simulink model "spring_mass_model_01"  (R2014a)
settings: Solver=FixedStepDiscrete  StartTime=0.0  StopTime=inf  FixedStep=sample_time  RelTol=1e-3
values from neighbouring files (symbols this model uses):
  g = g_real    (= 9.803)    [max_motor_torques.m]
  l0_leg = 0.97    [max_motor_torques.m]
  l0_virtual = sqrt(d^2+l0_leg^2-2*d*l0_leg*cos(phi0))    [max_motor_torques.m]
undefined symbols (not defined in the file or in its folder): alpha_apex, alpha_max, alpha_min, boom_mount_angle, c_energy, contact_threshold, control_start_time, d_y_boom_com_offset, d_y_boom_hip_offset, d_y_com, d_y_mount_to_com, desired_torso_angle, DiscIntNeverNeededParam, dt_thrust, dx_avg_desired, extra_leg_damping, F_thrust, fcut_contact, ff_energy_l, ff_energy_r, g_reduced, h_boom, i_limit_lateral, i_robot, initial_com_height, initial_dt, initial_dx, j_leg, j_rotor, j_segments, k0_virtual, k_placement, k_sea, kd_flight, kd_lateral, kd_leg_angle, kd_motor, kd_raibert, kd_torso, ki_lateral, kp_flight_max, kp_flight_min, kp_lateral, kp_leg_angle, kp_motor, kp_raibert, kp_torso, l0_max_angle_error, l0_min_angle_error, l0_min_flight_time, l_boom, l_boom_projected, l_max, l_min, l_retract_escape, l_retract_swing, l_seg, lambda1, lambda2, lateral_offset ... (+33)
libraries: simulink x22, simulink_extras x2
(part 2 of 3)

== system spring_mass_model_01/Control/Behavior Control/Contact Estimation/Contact Time ==
  Enable : EnablePort  StatesWhenEnabling=reset  ShowOutputPort=on
  Constant : Constant
  Discrete-Time Integrator : DiscreteIntegrator  IntegratorMethod=Accumulation: Forward Euler  gainval=sample_time  ExternalReset=rising  SampleTime=sample_time  ICPrevOutput=DiscIntNeverNeededParam  ICPrevScaledInput=DiscIntNeverNeededParam
  ts [s] : Outport  InitialOutput=[0]
  wires:
  Constant/1 -> Discrete-Time Integrator/1
  Enable/1 -> Discrete-Time Integrator/2
  Discrete-Time Integrator/1 -> ts [s]/1

== system spring_mass_model_01/Control/Behavior Control/Contact Estimation/Last Contact Time ==
  ts [s] : Inport
  Trigger : TriggerPort  TriggerType=falling  PortDimensions=1
  Ts [s] : Outport  InitialOutput=[initial_dt]
  wires:
  ts [s]/1 -> Ts [s]/1

== system spring_mass_model_01/Control/Behavior Control/Contact Estimation/Leg Torque Measurements ==
  q : Inport
  Right/Left Stance [1/0] : Inport  Port=2
  Spring Stiffness3 : Gain  Gain=k_sea(1)
  Spring Stiffness4 : Gain  Gain=k_sea(3)
  Spring Stiffness5 : Gain  Gain=k_sea(2)
  Spring Stiffness6 : Gain  Gain=k_sea(4)
  Sum{1..3,6} (4 alike) : Sum  Inputs=-+|
  Switch : Switch  Criteria=u2 ~= 0
  Switch1 : Switch  Criteria=u2 ~= 0
  backGearL : Selector  InputPortWidth=13  Indices=[6]
  backGearR : Selector  InputPortWidth=13  Indices=[2]
  backJointL : Selector  InputPortWidth=13  Indices=[5]
  backJointR : Selector  InputPortWidth=13  Indices=[1]
  frontGearL : Selector  InputPortWidth=13  Indices=[8]
  frontGearR : Selector  InputPortWidth=13  Indices=[4]
  frontJointL : Selector  InputPortWidth=13  Indices=[7]
  frontJointR : Selector  InputPortWidth=13  Indices=[3]
  Back [Nm] : Outport
  Front [Nm] : Outport  Port=2
  wires:
  Spring Stiffness6/1 -> Switch/3
  Spring Stiffness5/1 -> Switch/1
  Spring Stiffness4/1 -> Switch1/3
  Spring Stiffness3/1 -> Switch1/1
  q/1 -> backJointR/1, frontGearL/1, frontJointL/1, frontGearR/1, frontJointR/1, backGearL/1, backJointL/1, backGearR/1
  backGearR/1 -> Sum6/2
  frontJointR/1 -> Sum1/1
  frontGearR/1 -> Sum1/2
  backJointR/1 -> Sum6/1
  Switch/1 -> Front [Nm]/1
  Sum1/1 -> Spring Stiffness5/1
  Sum6/1 -> Spring Stiffness3/1
  backGearL/1 -> Sum2/2
  frontJointL/1 -> Sum3/1
  frontGearL/1 -> Sum3/2
  backJointL/1 -> Sum2/1
  Switch1/1 -> Back [Nm]/1
  Sum2/1 -> Spring Stiffness4/1
  Sum3/1 -> Spring Stiffness6/1
  Right/Left Stance [1/0]/1 -> Switch/2, Switch1/2

== system spring_mass_model_01/Control/Behavior Control/Contact Estimation/Vertical Spring Force ==
  theta [rad] : Inport
  phi [rad] : Inport  Port=2
  Force [N] : Inport  Port=3
  Gain : Gain  Gain=-1
  Product : Product
  Sum : Sum  Inputs=++|
  Trigonometric Function : Trigonometry  Operator=cos
  Vertical Force [N] : Outport
  wires:
  Force [N]/1 -> Product/1
  phi [rad]/1 -> Sum/2
  theta [rad]/1 -> Sum/1
  Trigonometric Function/1 -> Product/2
  Product/1 -> Gain/1
  Sum/1 -> Trigonometric Function/1
  Gain/1 -> Vertical Force [N]/1

== system spring_mass_model_01/Control/Behavior Control/Lateral PID Control/Lateral Hip PID ==
  position_error : Inport
  velocity_error : Inport  Port=2
  Discrete-Time Integrator : DiscreteIntegrator  IntegratorMethod=Integration: Trapezoidal  SampleTime=sample_time  LimitOutput=on  UpperSaturationLimit=i_limit_lateral  LowerSaturationLimit=-i_limit_lateral  ICPrevOutput=DiscIntNeverNeededParam  ICPrevScaledInput=DiscIntNeverNeededParam
  Sum : Sum  Inputs=+++
  kd_lateral : Gain  Description=xPCTag(1)=kd_lateral;  Gain=kd_lateral
  ki_lateral : Gain  Description=xPCTag(1)=ki_lateral;  Gain=ki_lateral
  kp_lateral : Gain  Description=xPCTag(1)=kp_lateral;  Gain=kp_lateral
  out : Outport
  wires:
  velocity_error/1 -> kd_lateral/1
  Discrete-Time Integrator/1 -> Sum/3
  ki_lateral/1 -> Discrete-Time Integrator/1
  kp_lateral/1 -> Sum/2
  position_error/1 -> ki_lateral/1, kp_lateral/1
  Sum/1 -> out/1
  kd_lateral/1 -> Sum/1

== system spring_mass_model_01/Control/Behavior Control/Lateral PID Control/spherical_correction_angle ==
  q_cmu : Inport
  Selector : Selector  InputPortWidth=13  Indices=[11]
  Sum1 : Sum  Inputs=|+-
  Terminator2 : Terminator
  boom_mount_angle : Constant  Value=boom_mount_angle
  lateral_correction : Gain  Gain=180/pi
  lateral_correction [rad] : Outport
  wires:
  Sum1/1 -> lateral_correction/1, lateral_correction [rad]/1
  Selector/1 -> Sum1/1  "qBoomRoll"
  q_cmu/1 -> Selector/1
  boom_mount_angle/1 -> Sum1/2
  lateral_correction/1 -> Terminator2/1

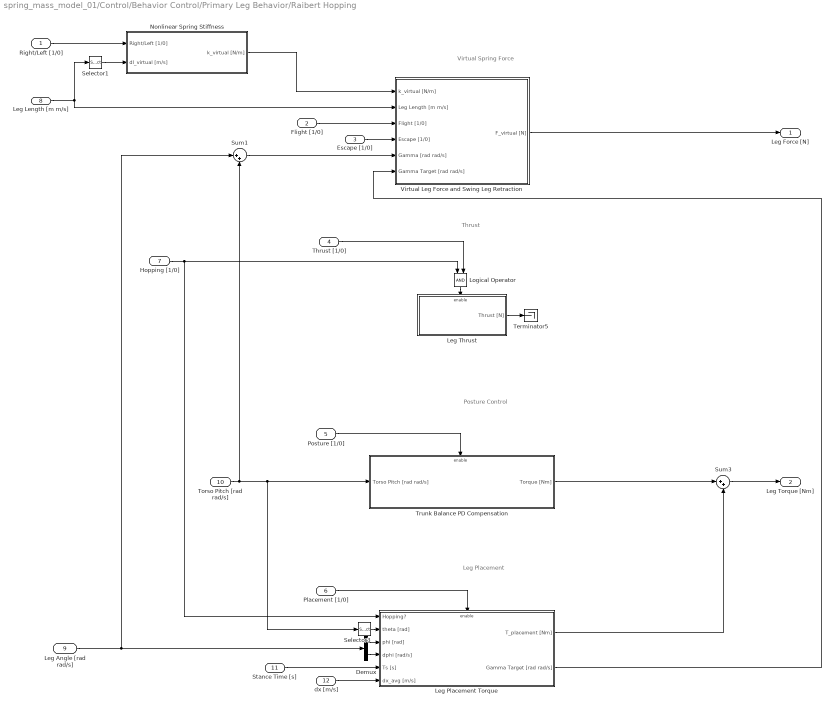
== system spring_mass_model_01/Control/Behavior Control/Primary Leg Behavior/Raibert Hopping ==
  note: Virtual Spring Force
  note: Thrust
  note: Posture Control
  note: Leg Placement
  Right/Left [1/0] : Inport
  Flight [1/0] : Inport  Port=2
  Escape [1/0] : Inport  Port=3
  Thrust [1/0] : Inport  Port=4
  Posture [1/0] : Inport  Port=5
  Placement [1/0] : Inport  Port=6
  Hopping [1/0] : Inport  Port=7
  Leg Length [m m/s] : Inport  Port=8
  Leg Angle [rad rad/s] : Inport  Port=9
  Torso Pitch [rad rad/s] : Inport  Port=10
  Stance Time [s] : Inport  Port=11
  dx [m/s] : Inport  Port=12
  Demux : Demux  Outputs=2
  Leg Placement Torque : Subsystem
  Leg Thrust : Subsystem
  Logical Operator : Logic  IconShape=distinctive  AllPortsSameDT=off  OutDataTypeStr=boolean
  Nonlinear Spring Stiffness : Subsystem
  Selector1 : Selector  InputPortWidth=2  Indices=[2]
  Selector3 : Selector  InputPortWidth=2  Indices=[1]
  Sum1 : Sum  Inputs=|++
  Sum3 : Sum  Inputs=|++
  Terminator5 : Terminator
  Trunk Balance PD Compensation : Subsystem
  Virtual Leg Force and Swing Leg Retraction : Subsystem
  Leg Force [N] : Outport
  Leg Torque [Nm] : Outport  Port=2
  wires:
  Sum3/1 -> Leg Torque [Nm]/1
  Logical Operator/1 -> Leg Thrust/Enable
  Trunk Balance PD Compensation/1(Torque [Nm]) -> Sum3/1
  Leg Placement Torque/1(T_placement [Nm]) -> Sum3/2
  Stance Time [s]/1 -> Leg Placement Torque/5(Ts [s])
  dx [m/s]/1 -> Leg Placement Torque/6(dx_avg [m/s])
  Escape [1/0]/1 -> Virtual Leg Force and Swing Leg Retraction/4(Escape [1/0])
  Thrust [1/0]/1 -> Logical Operator/2
  Leg Length [m m/s]/1 -> Virtual Leg Force and Swing Leg Retraction/2(Leg Length [m m/s]), Selector1/1
  Posture [1/0]/1 -> Trunk Balance PD Compensation/Enable
  Torso Pitch [rad rad/s]/1 -> Trunk Balance PD Compensation/1(Torso Pitch [rad rad/s]), Selector3/1, Sum1/2
  Selector3/1 -> Leg Placement Torque/2(theta [rad])
  Placement [1/0]/1 -> Leg Placement Torque/Enable
  Flight [1/0]/1 -> Virtual Leg Force and Swing Leg Retraction/3(Flight [1/0])
  Hopping [1/0]/1 -> Logical Operator/1, Leg Placement Torque/1(Hopping?)
  Demux/2 -> Leg Placement Torque/4(dphi [rad/s])
  Demux/1 -> Leg Placement Torque/3(phi [rad])
  Selector1/1 -> Nonlinear Spring Stiffness/2(dl_virtual [m/s])
  Right/Left [1/0]/1 -> Nonlinear Spring Stiffness/1(Right/Left [1/0])
  Leg Angle [rad rad/s]/1 -> Sum1/1, Demux/1
  Sum1/1 -> Virtual Leg Force and Swing Leg Retraction/5(Gamma [rad rad/s])
  Leg Placement Torque/2(Gamma Target [rad rad/s]) -> Virtual Leg Force and Swing Leg Retraction/6(Gamma Target [rad rad/s])
  Nonlinear Spring Stiffness/1(k_virtual [N/m]) -> Virtual Leg Force and Swing Leg Retraction/1(k_virtual [N/m])
  Virtual Leg Force and Swing Leg Retraction/1(F_virtual [N]) -> Leg Force [N]/1
  Leg Thrust/1(Thrust [N]) -> Terminator5/1

== system spring_mass_model_01/Control/Behavior Control/Primary Leg Behavior/SMM 01 ==
  note: Swing
  note: Stance
  Right/Left [1/0] : Inport
  Escape [1/0] : Inport  Port=2
  Posture [1/0] : Inport  Port=3
  Placement [1/0] : Inport  Port=4
  Primary Leg Angle [rad rad/s] : Inport  Port=5
  Primary Leg Length [m m/s] : Inport  Port=6
  Torso Pitch [rad rad/s] : Inport  Port=7
  Virtual Spring Length [m m/s] : Inport  Port=8
  Apex Time [s] : Inport  Port=9
  System Energy [J] : Inport  Port=10
  Primary Back Gear [rad rad/s] : Inport  Port=11
  Primary Front Gear [rad rad/s] : Inport  Port=12
  Primary w [m] : Inport  Port=13
  Logical Operator : Logic  Operator=NOT  AllPortsSameDT=off  OutDataTypeStr=boolean
  Primary Stance Phase : Subsystem
  Primary Swing Phase : Subsystem
  Leg Force [Nm] : Outport
  Leg Torque [Nm] : Outport  Port=2
  Back/Front Motor Torque [Nm Nm] : Outport  Port=3
  Primary Force or Position Control [1/0] : Outport  Port=4  OutDataTypeStr=boolean
  wires:
  Torso Pitch [rad rad/s]/1 -> Primary Stance Phase/2(Torso Pitch [rad rad/s]), Primary Swing Phase/4(Torso Pitch [rad rad/s])
  Primary Leg Length [m m/s]/1 -> Primary Stance Phase/1(Primary Leg Length [m m/s]), Primary Swing Phase/2(Primary Leg Length [m m/s])
  Right/Left [1/0]/1 -> Primary Swing Phase/8(Right/Left Primary [1/0]), Primary Stance Phase/4(Right/Left Primary [1/0])
  Placement [1/0]/1 -> Logical Operator/1
  Apex Time [s]/1 -> Primary Swing Phase/5(Time of Apex [s])
  Primary Back Gear [rad rad/s]/1 -> Primary Swing Phase/6(Primary Back Gear [rad rad/s])
  Primary Front Gear [rad rad/s]/1 -> Primary Swing Phase/7(Primary Front Gear [rad rad/s])
  Primary Swing Phase/1(Back/Front Motor Torque Command [Nm Nm]) -> Back/Front Motor Torque [Nm Nm]/1
  Primary Leg Angle [rad rad/s]/1 -> Primary Stance Phase/8(Primary Leg Angle [rad rad/s]), Primary Swing Phase/3(Primary Leg Angle [rad rad/s])
  Posture [1/0]/1 -> Primary Stance Phase/3(Enable Posture Control [1/0])
  System Energy [J]/1 -> Primary Stance Phase/5(System Energy [J])
  Virtual Spring Length [m m/s]/1 -> Primary Stance Phase/6(Virtual Spring Length [m m/s])
  Escape [1/0]/1 -> Primary Swing Phase/1(Escape [1/0])
  Primary Stance Phase/1(Leg Torque Command [Nm]) -> Leg Torque [Nm]/1
  Primary Stance Phase/2(Leg Force Command [Nm]) -> Leg Force [Nm]/1
  Logical Operator/1 -> Primary Force or Position Control [1/0]/1
  Primary w [m]/1 -> Primary Stance Phase/7(Primary w [m])

== system spring_mass_model_01/Control/Behavior Control/Secondary Leg Behavior/Back//Front Motor PD ==
  Desired Position [rad] [back front] : Inport
  Desired Velocity [rad/s] [back front] : Inport  Port=2
  Desired Acceleration [rad/s^2] [back front] : Inport  Port=3
  Measured Position [rad] [back front] : Inport  Port=4
  Measured Velocity [rad/s] [back front] : Inport  Port=5
  Right/Left Leg [1/0] : Inport  Port=6
  Friction Compensation : Subsystem
  Product : Product
  Sum1 : Sum  Inputs=|++
  Sum2 : Sum  Inputs=|++
  Sum7 : Sum  Inputs=|+-
  Sum8 : Sum  Inputs=|+-
  Sum9 : Sum
  Switch : Switch  Criteria=u2 ~= 0
  kd : Gain  Gain=kd_motor
  kp : Gain  Gain=kp_motor
  left_inertias : Constant  Value=j_segments(3:4)
  right_inertias : Constant  Value=j_segments(1:2)
  Commanded Torque [Nm] [back front] : Outport
  wires:
  Desired Velocity [rad/s] [back front]/1 -> Sum8/1, Friction Compensation/2(Commanded Velocity [rad/s] [back front])
  Friction Compensation/1(Friction Compensation [Nm]) -> Sum2/2
  Sum2/1 -> Commanded Torque [Nm] [back front]/1
  Switch/1 -> Product/2
  left_inertias/1 -> Switch/3
  right_inertias/1 -> Switch/1
  Right/Left Leg [1/0]/1 -> Switch/2, Friction Compensation/1(Right/Left [1/0])
  Product/1 -> Sum1/2
  Desired Acceleration [rad/s^2] [back front]/1 -> Product/1
  Sum1/1 -> Sum2/1
  Measured Velocity [rad/s] [back front]/1 -> Sum8/2
  kd/1 -> Sum9/2
  Desired Position [rad] [back front]/1 -> Sum7/1
  Sum8/1 -> kd/1
  Sum9/1 -> Sum1/1
  Measured Position [rad] [back front]/1 -> Sum7/2
  Sum7/1 -> kp/1
  kp/1 -> Sum9/1

== system spring_mass_model_01/Control/Behavior Control/Velocity Estimation/Recursive Moving Average ==
  Velocity [m/s] : Inport
  Delay : Delay  DelayLength=velocity_avg_samples  InitialCondition=0  UseCircularBuffer=on  SampleTime=sample_time
  Gain : Gain  Gain=1/velocity_avg_samples
  Sum : Sum  Inputs=-++
  Unit Delay : UnitDelay  SampleTime=sample_time
  Average Velocity [m/s] : Outport
  wires:
  Velocity [m/s]/1 -> Delay/1, Sum/2
  Sum/1 -> Unit Delay/1, Gain/1
  Delay/1 -> Sum/1
  Gain/1 -> Average Velocity [m/s]/1
  Unit Delay/1 -> Sum/3

== system spring_mass_model_01/Control/Behavior Control/Velocity Estimation/Signal During Escape ==
  signal : Inport
  time : Inport  Port=2
  Enable : EnablePort
  signal at escape : Outport
  time at escape : Outport  Port=2
  wires:
  signal/1 -> signal at escape/1
  time/1 -> time at escape/1

== system spring_mass_model_01/Control/Behavior Control/Velocity Estimation/Takeoff ==
  contact : Inport
  Compare To Constant : simulink/Logic and Bit Operations/Compare To Constant  relop=<=  const=TO_threshold  OutDataTypeStr=boolean
  Compare To Constant1 : simulink/Logic and Bit Operations/Compare To Constant  relop=>  const=TO_threshold  OutDataTypeStr=boolean
  Logical Operator : Logic  AllPortsSameDT=off  OutDataTypeStr=boolean
  Unit Delay1 : UnitDelay  SampleTime=sample_time
  takeoff : Outport
  wires:
  Compare To Constant1/1 -> Logical Operator/1
  Compare To Constant/1 -> Logical Operator/2
  contact/1 -> Compare To Constant/1, Unit Delay1/1
  Logical Operator/1 -> takeoff/1
  Unit Delay1/1 -> Compare To Constant1/1

== system spring_mass_model_01/Control/Behavior Control/Velocity Estimation/Takeoff Velocity ==
  Leg Length [m m/s] : Inport
  Leg Angle [rad rad/s] : Inport  Port=2
  Torso Pitch [rad rad/s] : Inport  Port=3
  Enable : EnablePort
  Demux2 : Demux  Outputs=2
  Demux3 : Demux  Outputs=2
  Demux4 : Demux  Outputs=2
  vertical_velocity : MATLAB Function  TreatAsAtomicUnit=on
  y_TO [m] : Outport  InitialOutput=[initial_com_height]
  dx_TO [m/s] : Outport  Port=2  InitialOutput=[initial_dx]
  dy_TO [m/s] : Outport  Port=3  InitialOutput=[0]
  wires:
  Demux2/1 -> vertical_velocity/1(l)
  Leg Length [m m/s]/1 -> Demux2/1
  Demux4/1 -> vertical_velocity/5(qPitch)
  Torso Pitch [rad rad/s]/1 -> Demux4/1
  Demux3/2 -> vertical_velocity/4(dphi)
  Demux3/1 -> vertical_velocity/3(phi)
  Leg Angle [rad rad/s]/1 -> Demux3/1
  Demux4/2 -> vertical_velocity/6(dqPitch)
  Demux2/2 -> vertical_velocity/2(dl)
  vertical_velocity/1(y) -> y_TO [m]/1
  vertical_velocity/2(dx) -> dx_TO [m/s]/1
  vertical_velocity/3(dy) -> dy_TO [m/s]/1

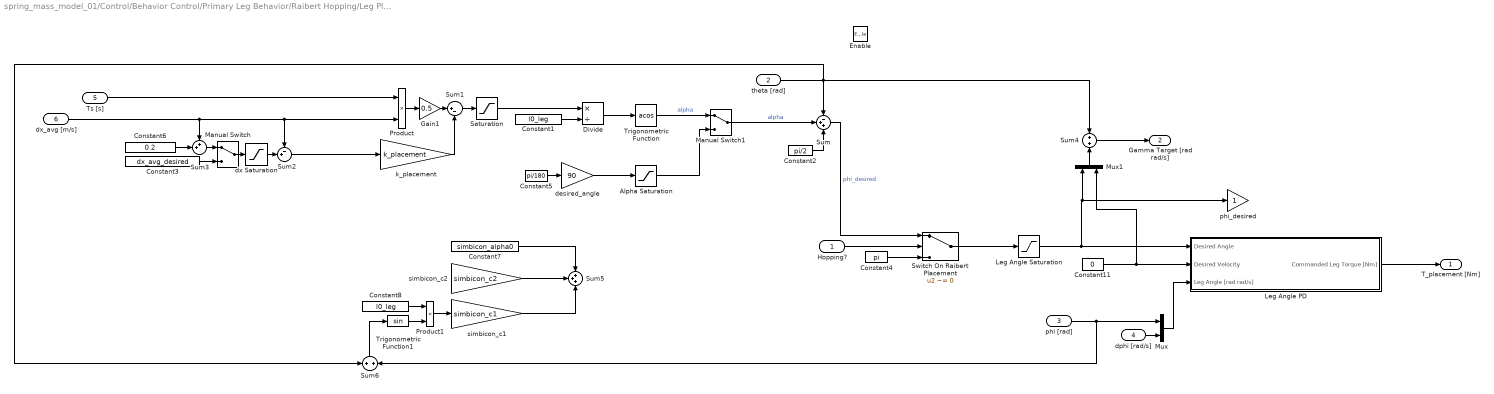
== system spring_mass_model_01/Control/Behavior Control/Primary Leg Behavior/Raibert Hopping/Leg Placement Torque ==
  Hopping? : Inport
  theta [rad] : Inport  Port=2
  phi [rad] : Inport  Port=3
  dphi [rad/s] : Inport  Port=4
  Ts [s] : Inport  Port=5
  dx_avg [m/s] : Inport  Port=6
  Enable : EnablePort  StatesWhenEnabling=reset
  Alpha Saturation : Saturate  UpperLimit=alpha_max  LowerLimit=alpha_min
      settings: AttributesFormatString=Hi: %<UpperLimit>\nLo: %<LowerLimit>
  Constant1 : Constant  Value=l0_leg
  Constant11 : Constant  Value=0
  Constant2 : Constant  Value=pi/2
  Constant3 : Constant  Value=dx_avg_desired
  Constant4 : Constant  Value=pi
  Constant5 : Constant  Value=pi/180
  Constant6 : Constant  Value=0.2
  Constant7 : Constant  Value=simbicon_alpha0
  Constant8 : Constant  Value=l0_leg
  Divide : Product  Inputs=*/
  Gain1 : Gain  Gain=0.5
  Leg Angle PD : Subsystem
  Leg Angle Saturation : Saturate  UpperLimit=max_leg_angle  LowerLimit=min_leg_angle
      settings: AttributesFormatString=Hi: %<UpperLimit>\nLo: %<LowerLimit>
  Manual Switch : ManualSwitch
  Manual Switch1 : ManualSwitch
  Mux : Mux  Inputs=2
  Mux1 : Mux  Inputs=2
  Product : Product
  Product1 : Product
  Saturation : Saturate  UpperLimit=x_limit  LowerLimit=-x_limit
      settings: AttributesFormatString=Hi: %<UpperLimit>\nLo: %<LowerLimit>
  Sum : Sum  Inputs=-++
  Sum1 : Sum  Inputs=|+-
  Sum2 : Sum  Inputs=-+|
  Sum3 : Sum  Inputs=++|
  Sum4 : Sum  Inputs=+|+
  Sum5 : Sum  Inputs=+++
  Sum6 : Sum  Inputs=+|+
  Switch On Raibert Placement : Switch  Criteria=u2 ~= 0
  Trigonometric Function : Trigonometry  Operator=acos
  Trigonometric Function1 : Trigonometry
  desired_angle : Gain  Gain=90
  dx Saturation : Saturate  UpperLimit=dx_avg_desired  LowerLimit=0
      settings: AttributesFormatString=Hi: %<UpperLimit>\nLo: %<LowerLimit>
  k_placement : Gain  Gain=k_placement
  phi_desired : Gain
  simbicon_c1 : Gain  Gain=simbicon_c1
  simbicon_c2 : Gain  Gain=simbicon_c2
  T_placement [Nm] : Outport  OutputWhenDisabled=reset  InitialOutput=[0]
  Gamma Target [rad rad/s] : Outport  Port=2  OutputWhenDisabled=reset  InitialOutput=[0]
  wires:
  Sum3/1 -> Manual Switch/1
  Constant6/1 -> Sum3/2
  dx_avg [m/s]/1 -> Product/2, Sum2/1, Sum3/1
  Constant3/1 -> Manual Switch/2
  Manual Switch/1 -> dx Saturation/1
  Switch On Raibert Placement/1 -> Leg Angle Saturation/1
  Constant5/1 -> desired_angle/1
  Leg Angle Saturation/1 -> Leg Angle PD/1(Desired Angle), phi_desired/1, Mux1/1
  Hopping?/1 -> Switch On Raibert Placement/2
  Constant4/1 -> Switch On Raibert Placement/3
  dx Saturation/1 -> Sum2/2
  k_placement/1 -> Sum1/2
  Sum1/1 -> Saturation/1
  Sum/1 -> Switch On Raibert Placement/1  "phi_desired"
  theta [rad]/1 -> Sum/1, Sum6/1, Sum4/1
  Constant2/1 -> Sum/3
  Manual Switch1/1 -> Sum/2  "alpha"
  Divide/1 -> Trigonometric Function/1
  Constant1/1 -> Divide/2
  Saturation/1 -> Divide/1
  Gain1/1 -> Sum1/1
  Product/1 -> Gain1/1
  Ts [s]/1 -> Product/1
  dphi [rad/s]/1 -> Mux/2
  phi [rad]/1 -> Sum6/2, Mux/1
  Leg Angle PD/1(Commanded Leg Torque [Nm]) -> T_placement [Nm]/1
  Mux/1 -> Leg Angle PD/3(Leg Angle [rad rad/s])
  Constant11/1 -> Mux1/2, Leg Angle PD/2(Desired Velocity)
  Sum4/1 -> Gamma Target [rad rad/s]/1
  Mux1/1 -> Sum4/2
  Trigonometric Function/1 -> Manual Switch1/1  "alpha"
  Constant7/1 -> Sum5/1
  simbicon_c1/1 -> Sum5/3
  simbicon_c2/1 -> Sum5/2
  Trigonometric Function1/1 -> Product1/2
  Product1/1 -> simbicon_c1/1
  Sum2/1 -> k_placement/1
  Constant8/1 -> Product1/1
  Sum6/1 -> Trigonometric Function1/1
  Alpha Saturation/1 -> Manual Switch1/2
  desired_angle/1 -> Alpha Saturation/1

== system spring_mass_model_01/Control/Behavior Control/Primary Leg Behavior/Raibert Hopping/Leg Thrust ==
  Enable : EnablePort  StatesWhenEnabling=reset  ShowOutputPort=on
  F_thrust : Gain  Gain=F_thrust
  Thrust Timer : Subsystem
  thrust period? : simulink/Logic and Bit Operations/Compare To Constant  relop=<=  const=dt_thrust  OutDataTypeStr=uint8
  Thrust [N] : Outport  OutputWhenDisabled=reset  InitialOutput=[0]
  wires:
  thrust period?/1 -> F_thrust/1
  Enable/1 -> Thrust Timer/Enable
  Thrust Timer/1(timer [s]) -> thrust period?/1
  F_thrust/1 -> Thrust [N]/1

== system spring_mass_model_01/Control/Behavior Control/Primary Leg Behavior/Raibert Hopping/Nonlinear Spring Stiffness ==
  Right/Left [1/0] : Inport
  dl_virtual [m/s] : Inport  Port=2
  E_target1 : Constant  Value=ff_energy_r
  E_target2 : Constant  Value=ff_energy_l
  Product : Product  Inputs=3
  Saturation : Saturate  UpperLimit=max_kp_raibert  LowerLimit=min_kp_raibert  ZeroCross=off
  Sum : Sum  Inputs=+|-
  Sum2 : Sum  Inputs=--|
  Switch1 : Switch  Criteria=u2 ~= 0
  c_energy : Constant  Value=c_energy
  c_energy1 : Constant  Value=raibert_energy_injection
  k0_virtual : Constant  Value=kp_raibert
  k_virtual [N/m] : Outport
  wires:
  Product/1 -> Sum/2
  Sum/1 -> Saturation/1
  Saturation/1 -> k_virtual [N/m]/1
  k0_virtual/1 -> Sum/1
  c_energy/1 -> Product/3
  dl_virtual [m/s]/1 -> Product/2
  E_target1/1 -> Switch1/1
  E_target2/1 -> Switch1/3
  Right/Left [1/0]/1 -> Switch1/2
  Switch1/1 -> Sum2/2
  c_energy1/1 -> Sum2/1
  Sum2/1 -> Product/1

== system spring_mass_model_01/Control/Behavior Control/Primary Leg Behavior/Raibert Hopping/Trunk Balance PD Compensation ==
  Torso Pitch [rad rad/s] : Inport
  Enable : EnablePort  StatesWhenEnabling=reset
  Constant2 : Constant  Value=0
  Demux : Demux  Outputs=2
  Derivative Gain : Gain  Gain=kd_torso
  Gain1 : Gain  Gain=-1
  Proportional Gain : Gain  Gain=kp_torso
  Reference Lean [rad] : Constant  Value=desired_torso_angle
  Sum1 : Sum  Inputs=|+-
  Sum4 : Sum  Inputs=|+-
  Sum5 : Sum
  Torque [Nm] : Outport  OutputWhenDisabled=reset  InitialOutput=[0]
  wires:
  Gain1/1 -> Torque [Nm]/1
  Sum1/1 -> Derivative Gain/1
  Proportional Gain/1 -> Sum5/1
  Derivative Gain/1 -> Sum5/2
  Torso Pitch [rad rad/s]/1 -> Demux/1
  Sum4/1 -> Proportional Gain/1
  Demux/1 -> Sum4/2
  Reference Lean [rad]/1 -> Sum4/1
  Constant2/1 -> Sum1/1
  Demux/2 -> Sum1/2
  Sum5/1 -> Gain1/1

== system spring_mass_model_01/Control/Behavior Control/Primary Leg Behavior/Raibert Hopping/Virtual Leg Force and Swing Leg Retraction ==
  k_virtual [N/m] : Inport
  Leg Length [m m/s] : Inport  Port=2
  Flight [1/0] : Inport  Port=3
  Escape [1/0] : Inport  Port=4
  Gamma [rad rad/s] : Inport  Port=5
  Gamma Target [rad rad/s] : Inport  Port=6
  Demux1 : Demux  Outputs=2
  Demux2 : Demux  Outputs=2
  Demux3 : Demux  Outputs=2
  Virtual Spring Force : MATLAB Function  TreatAsAtomicUnit=on
  F_virtual [N] : Outport
  wires:
  Virtual Spring Force/1(F_virtual) -> F_virtual [N]/1
  Flight [1/0]/1 -> Virtual Spring Force/5(flight)
  Demux1/1 -> Virtual Spring Force/8(l_spring)
  Leg Length [m m/s]/1 -> Demux1/1
  Demux1/2 -> Virtual Spring Force/9(dl_spring)
  Escape [1/0]/1 -> Virtual Spring Force/6(escape)
  k_virtual [N/m]/1 -> Virtual Spring Force/7(k_virtual)
  Demux2/1 -> Virtual Spring Force/1(gamma)
  Demux2/2 -> Virtual Spring Force/2(dgamma)
  Demux3/1 -> Virtual Spring Force/3(gamma_tgt)
  Demux3/2 -> Virtual Spring Force/4(dgamma_tgt)
  Gamma [rad rad/s]/1 -> Demux2/1
  Gamma Target [rad rad/s]/1 -> Demux3/1

== system spring_mass_model_01/Control/Behavior Control/Primary Leg Behavior/SMM 01/Primary Stance Phase ==
  note: Posture control loop
      | to prevent the torso
      | from falling over
  note: Command a virtual spring
      | force to match the SMM
      | using inverse dynamics
  note: Stance
  note: Modulate virtual spring
      | stiffness to regulate
      | energy during stance
  note: (alternatively: rotate the GRF vector in the inverse dynamics)
  Primary Leg Length [m m/s] : Inport
  Torso Pitch [rad rad/s] : Inport  Port=2
  Enable Posture Control [1/0] : Inport  Port=3
  Right/Left Primary [1/0] : Inport  Port=4
  System Energy [J] : Inport  Port=5
  Virtual Spring Length [m m/s] : Inport  Port=6
  Primary w [m] : Inport  Port=7
  Primary Leg Angle [rad rad/s] : Inport  Port=8
  E_target1 : Constant  Value=ff_energy_r
  E_target2 : Constant  Value=ff_energy_l
  Nonlinear Spring Stiffness : Subsystem
  Selector3 : Selector  InputPortWidth=2  Indices=[2]
  Sum3 : Sum  Inputs=|+-
  Sum4 : Sum  Inputs=-+|
  Switch1 : Switch  Criteria=u2 ~= 0
  Terminator : Terminator
  Terminator1 : Terminator
  Trunk Balance PD Compensation : Subsystem
  Virtual Leg Force and Swing Leg Retraction : Subsystem
  k_virtual : Gain
  target_energy : Constant  Value=target_energy
  Leg Torque Command [Nm] : Outport
  Leg Force Command [Nm] : Outport  Port=2
  wires:
  Switch1/1 -> Sum4/1
  System Energy [J]/1 -> Sum3/2
  k_virtual/1 -> Terminator1/1
  target_energy/1 -> Sum4/2
  Virtual Spring Length [m m/s]/1 -> Virtual Leg Force and Swing Leg Retraction/6(Virtual Spring Length [m m/s])
  Nonlinear Spring Stiffness/1(k_virtual [N/m]) -> k_virtual/1, Virtual Leg Force and Swing Leg Retraction/1(k_virtual [N/m])
  Sum3/1 -> Nonlinear Spring Stiffness/1(Energy Error [J])
  Enable Posture Control [1/0]/1 -> Trunk Balance PD Compensation/Enable
  Selector3/1 -> Nonlinear Spring Stiffness/2(dl_virtual [m/s])
  E_target1/1 -> Switch1/1
  Sum4/1 -> Sum3/1
  E_target2/1 -> Switch1/3
  Torso Pitch [rad rad/s]/1 -> Trunk Balance PD Compensation/1(Torso Pitch [rad rad/s]), Virtual Leg Force and Swing Leg Retraction/4(Torso Pitch [rad rad/s])
  Right/Left Primary [1/0]/1 -> Switch1/2
  Primary Leg Length [m m/s]/1 -> Selector3/1, Virtual Leg Force and Swing Leg Retraction/2(Leg Length [m m/s])
  Virtual Leg Force and Swing Leg Retraction/1(Leg Force [N]) -> Leg Force Command [Nm]/1
  Trunk Balance PD Compensation/1(Torque [Nm]) -> Terminator/1
  Primary w [m]/1 -> Virtual Leg Force and Swing Leg Retraction/5(Primary w [m])
  Primary Leg Angle [rad rad/s]/1 -> Virtual Leg Force and Swing Leg Retraction/3(Leg Angle [rad rad/s])
  Virtual Leg Force and Swing Leg Retraction/2(Leg Torque [Nm]) -> Leg Torque Command [Nm]/1

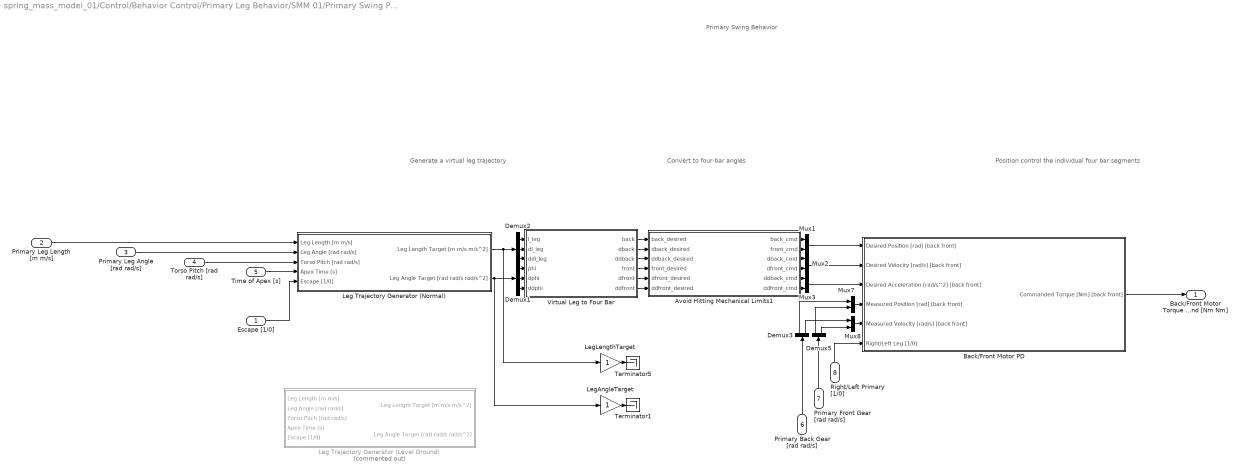
== system spring_mass_model_01/Control/Behavior Control/Primary Leg Behavior/SMM 01/Primary Swing Phase ==
  note: Generate a virtual
      | leg trajectory
  note: Position control the
      | individual four bar segments
  note: Primary Swing Behavior
  note: Convert to
      | four-bar angles
  Escape [1/0] : Inport
  Primary Leg Length [m m/s] : Inport  Port=2
  Primary Leg Angle [rad rad/s] : Inport  Port=3
  Torso Pitch [rad rad/s] : Inport  Port=4
  Time of Apex [s] : Inport  Port=5
  Primary Back Gear [rad rad/s] : Inport  Port=6
  Primary Front Gear [rad rad/s] : Inport  Port=7
  Right/Left Primary [1/0] : Inport  Port=8
  Avoid Hitting Mechanical Limits1 : MATLAB Function  TreatAsAtomicUnit=on
  Back/Front Motor PD : Subsystem
  Demux1 : Demux  Outputs=3
  Demux2 : Demux  Outputs=3
  Demux3 : Demux  Outputs=2
  Demux5 : Demux  Outputs=2
  Leg Trajectory Generator (Level Ground) : Subsystem  Commented=on
  Leg Trajectory Generator (Normal) : Subsystem
  LegAngleTarget : Gain
  LegLengthTarget : Gain
  Mux{1..3,7..8} (5 alike) : Mux  Inputs=2
  Terminator1 : Terminator
  Terminator5 : Terminator
  Virtual Leg to Four Bar : MATLAB Function  TreatAsAtomicUnit=on
  Back/Front Motor Torque Command [Nm Nm] : Outport
  wires:
  Leg Trajectory Generator (Normal)/2(Leg Angle Target [rad rad/s rad/s^2]) -> Demux1/1, LegAngleTarget/1
  Escape [1/0]/1 -> Leg Trajectory Generator (Normal)/5(Escape [1/0])
  Mux8/1 -> Back/Front Motor PD/5(Measured Velocity [rad/s] [back front])
  Demux5/2 -> Mux8/2
  Time of Apex [s]/1 -> Leg Trajectory Generator (Normal)/4(Apex Time [s])
  Virtual Leg to Four Bar/5(dfront) -> Avoid Hitting Mechanical Limits1/5(dfront_desired)
  Mux7/1 -> Back/Front Motor PD/4(Measured Position [rad] [back front])
  Mux1/1 -> Back/Front Motor PD/1(Desired Position [rad] [back front])
  Primary Leg Length [m m/s]/1 -> Leg Trajectory Generator (Normal)/1(Leg Length [m m/s])
  Primary Leg Angle [rad rad/s]/1 -> Leg Trajectory Generator (Normal)/2(Leg Angle [rad rad/s])
  Right/Left Primary [1/0]/1 -> Back/Front Motor PD/6(Right/Left Leg [1/0])
  Torso Pitch [rad rad/s]/1 -> Leg Trajectory Generator (Normal)/3(Torso Pitch [rad rad/s])
  Demux3/2 -> Mux8/1
  Demux3/1 -> Mux7/1
  Virtual Leg to Four Bar/2(dback) -> Avoid Hitting Mechanical Limits1/2(dback_desired)
  Virtual Leg to Four Bar/4(front) -> Avoid Hitting Mechanical Limits1/4(front_desired)
  Virtual Leg to Four Bar/6(ddfront) -> Avoid Hitting Mechanical Limits1/6(ddfront_desired)
  Virtual Leg to Four Bar/3(ddback) -> Avoid Hitting Mechanical Limits1/3(ddback_desired)
  Avoid Hitting Mechanical Limits1/2(front_cmd) -> Mux1/2
  Virtual Leg to Four Bar/1(back) -> Avoid Hitting Mechanical Limits1/1(back_desired)
  Avoid Hitting Mechanical Limits1/1(back_cmd) -> Mux1/1
  Demux5/1 -> Mux7/2
  Back/Front Motor PD/1(Commanded Torque [Nm] [back front]) -> Back/Front Motor Torque Command [Nm Nm]/1
  Demux2/3 -> Virtual Leg to Four Bar/3(ddl_leg)
  Demux1/3 -> Virtual Leg to Four Bar/6(ddphi)
  Demux2/2 -> Virtual Leg to Four Bar/2(dl_leg)
  Demux1/1 -> Virtual Leg to Four Bar/4(phi)
  Demux1/2 -> Virtual Leg to Four Bar/5(dphi)
  Demux2/1 -> Virtual Leg to Four Bar/1(l_leg)
  Primary Front Gear [rad rad/s]/1 -> Demux5/1
  Primary Back Gear [rad rad/s]/1 -> Demux3/1
  Avoid Hitting Mechanical Limits1/3(dback_cmd) -> Mux2/1
  Avoid Hitting Mechanical Limits1/4(dfront_cmd) -> Mux2/2
  Avoid Hitting Mechanical Limits1/5(ddback_cmd) -> Mux3/1
  Avoid Hitting Mechanical Limits1/6(ddfront_cmd) -> Mux3/2
  Mux2/1 -> Back/Front Motor PD/2(Desired Velocity [rad/s] [back front])
  Mux3/1 -> Back/Front Motor PD/3(Desired Acceleration [rad/s^2] [back front])
  LegLengthTarget/1 -> Terminator5/1
  Leg Trajectory Generator (Normal)/1(Leg Length Target [m m/s m/s^2]) -> Demux2/1, LegLengthTarget/1
  LegAngleTarget/1 -> Terminator1/1

== system spring_mass_model_01/Control/Behavior Control/Secondary Leg Behavior/Back//Front Motor PD/Friction Compensation ==
  Right/Left [1/0] : Inport
  Commanded Velocity [rad/s] [back front] : Inport  Port=2
  Product : Product
  Sign : Signum
  Sum1 : Sum
  Switch : Switch  Criteria=u2 ~= 0
  Switch1 : Switch  Criteria=u2 ~= 0
  coulomb_friction_left : Constant  Value=sea_coulomb_friction(3:4)
  coulomb_friction_right : Constant  Value=sea_coulomb_friction(1:2)
  offset_friction_left : Constant  Value=sea_offset_friction(3:4)
  offset_friction_right : Constant  Value=sea_offset_friction(1:2)
  Friction Compensation [Nm] : Outport
  wires:
  Sign/1 -> Product/1
  Switch1/1 -> Product/2
  coulomb_friction_left/1 -> Switch1/3
  coulomb_friction_right/1 -> Switch1/1
  offset_friction_left/1 -> Switch/3
  offset_friction_right/1 -> Switch/1
  Right/Left [1/0]/1 -> Switch/2, Switch1/2
  Product/1 -> Sum1/1
  Sum1/1 -> Friction Compensation [Nm]/1
  Switch/1 -> Sum1/2
  Commanded Velocity [rad/s] [back front]/1 -> Sign/1

== system spring_mass_model_01/Control/Behavior Control/Primary Leg Behavior/Raibert Hopping/Leg Placement Torque/Leg Angle PD ==
  Desired Angle : Inport
  Desired Velocity : Inport  Port=2
  Leg Angle [rad rad/s] : Inport  Port=3
  Demux1 : Demux  Outputs=2
  Sum7 : Sum  Inputs=|+-
  Sum8 : Sum  Inputs=|+-
  Sum9 : Sum
  kd_leg_angle : Gain  Gain=kd_leg_angle
  kp_leg_angle : Gain  Gain=kp_leg_angle
  Commanded Leg Torque [Nm] : Outport
  wires:
  kp_leg_angle/1 -> Sum9/1
  Sum7/1 -> kp_leg_angle/1
  Demux1/1 -> Sum7/2
  Sum9/1 -> Commanded Leg Torque [Nm]/1
  Desired Velocity/1 -> Sum8/1
  Sum8/1 -> kd_leg_angle/1
  Desired Angle/1 -> Sum7/1
  kd_leg_angle/1 -> Sum9/2
  Demux1/2 -> Sum8/2
  Leg Angle [rad rad/s]/1 -> Demux1/1

== system spring_mass_model_01/Control/Behavior Control/Primary Leg Behavior/Raibert Hopping/Leg Thrust/Thrust Timer ==
  Enable : EnablePort  StatesWhenEnabling=reset  ShowOutputPort=on
  Constant : Constant
  Discrete-Time Integrator : DiscreteIntegrator  IntegratorMethod=Accumulation: Forward Euler  gainval=sample_time  ExternalReset=rising  SampleTime=sample_time  ICPrevOutput=DiscIntNeverNeededParam  ICPrevScaledInput=DiscIntNeverNeededParam
  timer [s] : Outport  InitialOutput=[0]
  wires:
  Constant/1 -> Discrete-Time Integrator/1
  Enable/1 -> Discrete-Time Integrator/2
  Discrete-Time Integrator/1 -> timer [s]/1

== system spring_mass_model_01/Control/Behavior Control/Primary Leg Behavior/SMM 01/Primary Stance Phase/Nonlinear Spring Stiffness ==
  Energy Error [J] : Inport
  dl_virtual [m/s] : Inport  Port=2
  Product : Product  Inputs=3
  Saturation : Saturate  UpperLimit=max_k_virtual  LowerLimit=min_k_virtual  ZeroCross=off
  Sum : Sum  Inputs=+|-
  c_energy : Constant  Value=c_energy
  k0_virtual : Constant  Value=k0_virtual
  k_virtual [N/m] : Outport
  wires:
  Product/1 -> Sum/2
  Sum/1 -> Saturation/1
  Saturation/1 -> k_virtual [N/m]/1
  Energy Error [J]/1 -> Product/1
  k0_virtual/1 -> Sum/1
  c_energy/1 -> Product/3
  dl_virtual [m/s]/1 -> Product/2

== system spring_mass_model_01/Control/Behavior Control/Primary Leg Behavior/SMM 01/Primary Stance Phase/Trunk Balance PD Compensation ==
  Torso Pitch [rad rad/s] : Inport
  Enable : EnablePort  StatesWhenEnabling=reset
  Constant2 : Constant  Value=0
  Demux : Demux  Outputs=2
  Derivative Gain : Gain  Gain=kd_torso
  Gain1 : Gain  Gain=-1
  Proportional Gain : Gain  Gain=kp_torso
  Reference Lean [rad] : Constant  Value=desired_torso_angle
  Sum1 : Sum  Inputs=|+-
  Sum4 : Sum  Inputs=|+-
  Sum5 : Sum
  Torque [Nm] : Outport  OutputWhenDisabled=reset  InitialOutput=[0]
  wires:
  Gain1/1 -> Torque [Nm]/1
  Sum1/1 -> Derivative Gain/1
  Proportional Gain/1 -> Sum5/1
  Derivative Gain/1 -> Sum5/2
  Torso Pitch [rad rad/s]/1 -> Demux/1
  Sum4/1 -> Proportional Gain/1
  Demux/1 -> Sum4/2
  Reference Lean [rad]/1 -> Sum4/1
  Constant2/1 -> Sum1/1
  Demux/2 -> Sum1/2
  Sum5/1 -> Gain1/1

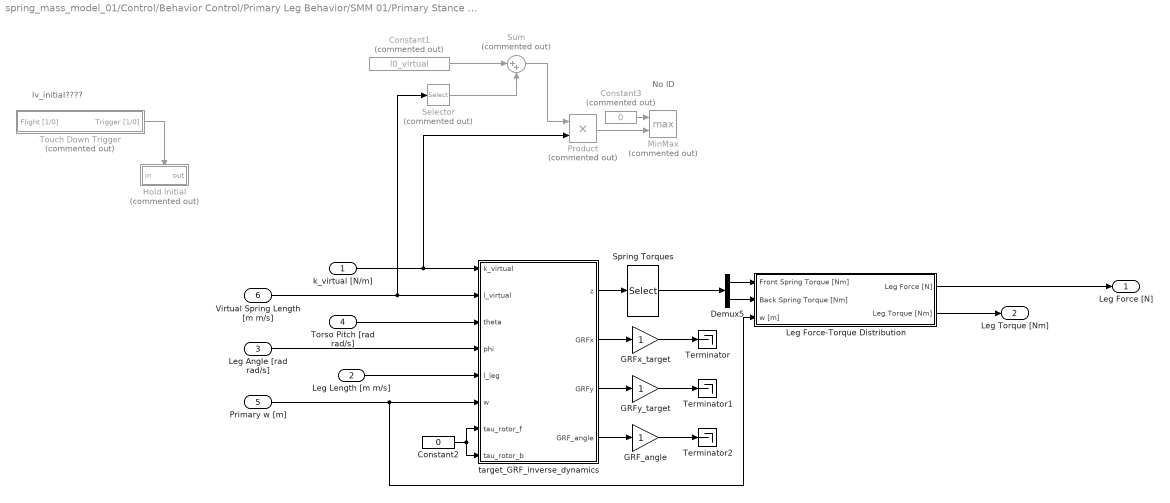
== system spring_mass_model_01/Control/Behavior Control/Primary Leg Behavior/SMM 01/Primary Stance Phase/Virtual Leg Force and Swing Leg Retraction ==
  note: No ID
  note: lv_initial????
  k_virtual [N/m] : Inport
  Leg Length [m m/s] : Inport  Port=2
  Leg Angle [rad rad/s] : Inport  Port=3
  Torso Pitch [rad rad/s] : Inport  Port=4
  Primary w [m] : Inport  Port=5
  Virtual Spring Length [m m/s] : Inport  Port=6
  Constant1 : Constant  Commented=on  Value=l0_virtual
  Constant2 : Constant  Value=0
  Constant3 : Constant  Commented=on  Value=0
  Demux5 : Demux  Outputs=2
  GRF_angle : Gain
  GRFx_target : Gain
  GRFy_target : Gain
  Hold Initial : Subsystem  Commented=on
  Leg Force-Torque Distribution : Subsystem
  MinMax : MinMax  Commented=on  Function=max  Inputs=2
  Product : Product  Commented=on
  Selector : Selector  Commented=on  InputPortWidth=2  Indices=[1]
  Spring Torques : Selector  InputPortWidth=7  Indices=[6 7]
  Sum : Sum  Commented=on  Inputs=|++
  Terminator : Terminator
  Terminator1 : Terminator
  Terminator2 : Terminator
  Touch Down Trigger : Subsystem  Commented=on
  target_GRF_inverse_dynamics : MATLAB Function  TreatAsAtomicUnit=on
  Leg Force [N] : Outport
  Leg Torque [Nm] : Outport  Port=2
  wires:
  Virtual Spring Length [m m/s]/1 -> Selector/1, target_GRF_inverse_dynamics/2(l_virtual)
  k_virtual [N/m]/1 -> Product/2, target_GRF_inverse_dynamics/1(k_virtual)
  Touch Down Trigger/1(Trigger [1/0]) -> Hold Initial/Trigger
  Leg Length [m m/s]/1 -> target_GRF_inverse_dynamics/5(l_leg)
  Constant2/1 -> target_GRF_inverse_dynamics/7(tau_rotor_f), target_GRF_inverse_dynamics/8(tau_rotor_b)
  target_GRF_inverse_dynamics/1(z) -> Spring Torques/1
  Demux5/2 -> Leg Force-Torque Distribution/2(Back Spring Torque [Nm])
  Demux5/1 -> Leg Force-Torque Distribution/1(Front Spring Torque [Nm])
  Spring Torques/1 -> Demux5/1
  Primary w [m]/1 -> Leg Force-Torque Distribution/3(w [m]), target_GRF_inverse_dynamics/6(w)
  Leg Force-Torque Distribution/2(Leg Torque [Nm]) -> Leg Torque [Nm]/1
  target_GRF_inverse_dynamics/2(GRFx) -> GRFx_target/1
  target_GRF_inverse_dynamics/3(GRFy) -> GRFy_target/1
  target_GRF_inverse_dynamics/4(GRF_angle) -> GRF_angle/1
  Torso Pitch [rad rad/s]/1 -> target_GRF_inverse_dynamics/3(theta)
  Leg Angle [rad rad/s]/1 -> target_GRF_inverse_dynamics/4(phi)
  GRFx_target/1 -> Terminator/1
  GRFy_target/1 -> Terminator1/1
  GRF_angle/1 -> Terminator2/1
  Constant1/1 -> Sum/1
  Selector/1 -> Sum/2
  Sum/1 -> Product/1
  Product/1 -> MinMax/2
  Constant3/1 -> MinMax/1
  Leg Force-Torque Distribution/1(Leg Force [N]) -> Leg Force [N]/1

== system spring_mass_model_01/Control/Behavior Control/Primary Leg Behavior/SMM 01/Primary Swing Phase/Back//Front Motor PD ==
  Desired Position [rad] [back front] : Inport
  Desired Velocity [rad/s] [back front] : Inport  Port=2
  Desired Acceleration [rad/s^2] [back front] : Inport  Port=3
  Measured Position [rad] [back front] : Inport  Port=4
  Measured Velocity [rad/s] [back front] : Inport  Port=5
  Right/Left Leg [1/0] : Inport  Port=6
  Friction Compensation : Subsystem
  Product : Product
  Sum1 : Sum  Inputs=|++
  Sum2 : Sum  Inputs=|++
  Sum7 : Sum  Inputs=|+-
  Sum8 : Sum  Inputs=|+-
  Sum9 : Sum
  Switch : Switch  Criteria=u2 ~= 0
  kd : Gain  Gain=kd_motor
  kp : Gain  Gain=kp_motor
  left_inertias : Constant  Value=j_segments(3:4)
  right_inertias : Constant  Value=j_segments(1:2)
  Commanded Torque [Nm] [back front] : Outport
  wires:
  Desired Velocity [rad/s] [back front]/1 -> Sum8/1, Friction Compensation/2(Commanded Velocity [rad/s] [back front])
  Friction Compensation/1(Friction Compensation [Nm]) -> Sum2/2
  Sum2/1 -> Commanded Torque [Nm] [back front]/1
  Switch/1 -> Product/2
  left_inertias/1 -> Switch/3
  right_inertias/1 -> Switch/1
  Right/Left Leg [1/0]/1 -> Switch/2, Friction Compensation/1(Right/Left [1/0])
  Product/1 -> Sum1/2
  Desired Acceleration [rad/s^2] [back front]/1 -> Product/1
  Sum1/1 -> Sum2/1
  Measured Velocity [rad/s] [back front]/1 -> Sum8/2
  kd/1 -> Sum9/2
  Desired Position [rad] [back front]/1 -> Sum7/1
  Sum8/1 -> kd/1
  Sum9/1 -> Sum1/1
  Measured Position [rad] [back front]/1 -> Sum7/2
  Sum7/1 -> kp/1
  kp/1 -> Sum9/1

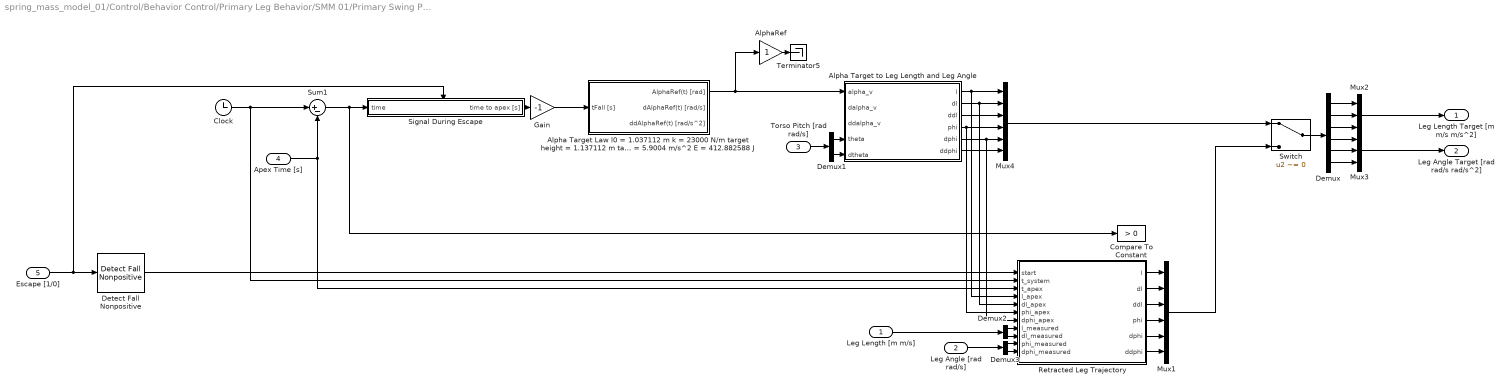
== system spring_mass_model_01/Control/Behavior Control/Primary Leg Behavior/SMM 01/Primary Swing Phase/Leg Trajectory Generator (Level Ground) ==
  Leg Length [m m/s] : Inport
  Leg Angle [rad rad/s] : Inport  Port=2
  Torso Pitch [rad rad/s] : Inport  Port=3
  Apex Time [s] : Inport  Port=4
  Escape [1/0] : Inport  Port=5
  Alpha Target Law l0 = 1.037112 m k = 23000 N/m target height = 1.137112 m target speed = 0.5 m/s m = 60.4120 kg g = 5.9004 m/s^2 E = 412.882588 J : Subsystem
  Alpha Target to Leg Length and Leg Angle : MATLAB Function  TreatAsAtomicUnit=on
  AlphaRef : Gain
  Clock : Clock
  Compare To Constant : simulink/Logic and Bit Operations/Compare To Constant  relop=>  const=0  OutDataTypeStr=boolean  ZeroCross=off
  Demux : Demux  Outputs=6
  Demux1 : Demux  Outputs=2
  Demux2 : Demux  Outputs=2
  Demux3 : Demux  Outputs=2
  Detect Fall Nonpositive : simulink/Logic and Bit Operations/Detect Fall Nonpositive  vinit=0  InputProcessing=Inherited  OutDataTypeStr=boolean
  Gain : Gain  Gain=-1
  Mux1 : Mux  Inputs=6
  Mux2 : Mux  Inputs=3
  Mux3 : Mux  Inputs=3
  Mux4 : Mux  Inputs=6
  Retracted Leg Trajectory : MATLAB Function  TreatAsAtomicUnit=on
  Signal During Escape : Subsystem
  Sum1 : Sum  Inputs=|+-
  Switch : Switch  Criteria=u2 ~= 0
  Terminator5 : Terminator
  Leg Length Target [m m/s m/s^2] : Outport
  Leg Angle Target [rad rad/s rad/s^2] : Outport  Port=2
  wires:
  Torso Pitch [rad rad/s]/1 -> Demux1/1
  Mux1/1 -> Switch/3
  Apex Time [s]/1 -> Retracted Leg Trajectory/3(t_apex), Sum1/2
  Clock/1 -> Retracted Leg Trajectory/2(t_system), Sum1/1
  Alpha Target Law l0 = 1.037112 m k = 23000 N/m target height = 1.137112 m target speed = 0.5 m/s m = 60.4120 kg g = 5.9004 m/s^2 E = 412.882588 J/1(AlphaRef(t) [rad]) -> AlphaRef/1, Alpha Target to Leg Length and Leg Angle/1(alpha_v)
  Sum1/1 -> Signal During Escape/1(time), Compare To Constant/1
  AlphaRef/1 -> Terminator5/1
  Retracted Leg Trajectory/1(l) -> Mux1/1
  Retracted Leg Trajectory/4(phi) -> Mux1/4
  Retracted Leg Trajectory/2(dl) -> Mux1/2
  Retracted Leg Trajectory/5(dphi) -> Mux1/5
  Escape [1/0]/1 -> Detect Fall Nonpositive/1, Signal During Escape/Enable
  Detect Fall Nonpositive/1 -> Retracted Leg Trajectory/1(start)
  Alpha Target to Leg Length and Leg Angle/4(phi) -> Retracted Leg Trajectory/6(phi_apex), Mux4/4
  Alpha Target to Leg Length and Leg Angle/3(ddl) -> Mux4/3
  Alpha Target to Leg Length and Leg Angle/5(dphi) -> Retracted Leg Trajectory/7(dphi_apex), Mux4/5
  Alpha Target to Leg Length and Leg Angle/6(ddphi) -> Mux4/6
  Alpha Target to Leg Length and Leg Angle/2(dl) -> Retracted Leg Trajectory/5(dl_apex), Mux4/2
  Alpha Target to Leg Length and Leg Angle/1(l) -> Retracted Leg Trajectory/4(l_apex), Mux4/1
  Switch/1 -> Demux/1
  Mux2/1 -> Leg Length Target [m m/s m/s^2]/1
  Mux3/1 -> Leg Angle Target [rad rad/s rad/s^2]/1
  Demux/6 -> Mux3/3
  Demux/5 -> Mux3/2
  Demux/4 -> Mux3/1
  Demux/3 -> Mux2/3
  Demux/2 -> Mux2/2
  Demux/1 -> Mux2/1
  Demux1/1 -> Alpha Target to Leg Length and Leg Angle/4(theta)
  Demux1/2 -> Alpha Target to Leg Length and Leg Angle/5(dtheta)
  Mux4/1 -> Switch/1
  Retracted Leg Trajectory/3(ddl) -> Mux1/3
  Retracted Leg Trajectory/6(ddphi) -> Mux1/6
  Demux2/1 -> Retracted Leg Trajectory/8(l_measured)
  Demux2/2 -> Retracted Leg Trajectory/9(dl_measured)
  Demux3/1 -> Retracted Leg Trajectory/10(phi_measured)
  Demux3/2 -> Retracted Leg Trajectory/11(dphi_measured)
  Leg Angle [rad rad/s]/1 -> Demux3/1
  Leg Length [m m/s]/1 -> Demux2/1
  Signal During Escape/1(time to apex [s]) -> Gain/1
  Gain/1 -> Alpha Target Law l0 = 1.037112 m k = 23000 N/m target height = 1.137112 m target speed = 0.5 m/s m = 60.4120 kg g = 5.9004 m/s^2 E = 412.882588 J/1(tFall [s])

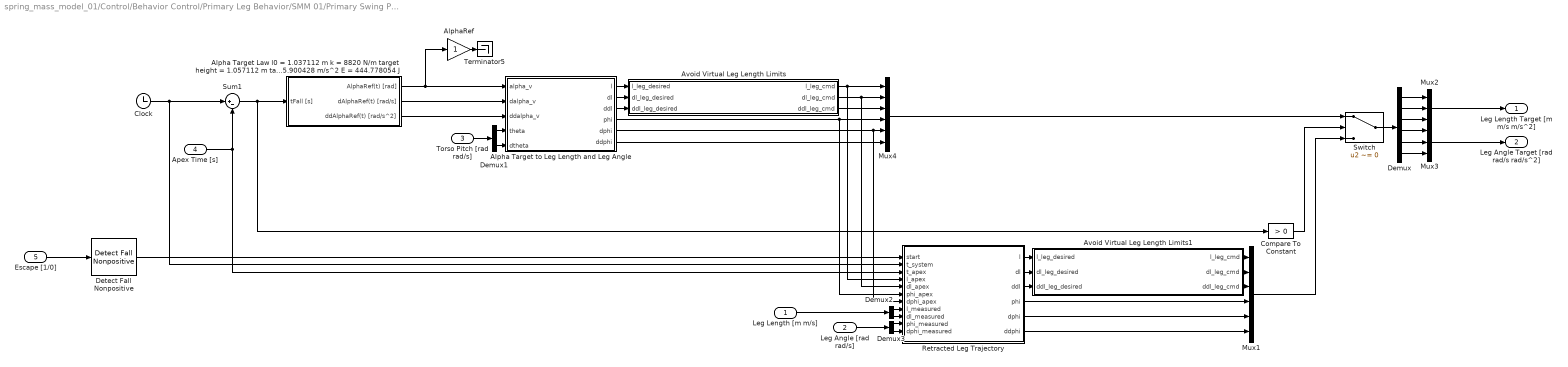
== system spring_mass_model_01/Control/Behavior Control/Primary Leg Behavior/SMM 01/Primary Swing Phase/Leg Trajectory Generator (Normal) ==
  Leg Length [m m/s] : Inport
  Leg Angle [rad rad/s] : Inport  Port=2
  Torso Pitch [rad rad/s] : Inport  Port=3
  Apex Time [s] : Inport  Port=4
  Escape [1/0] : Inport  Port=5
  Alpha Target Law l0 = 1.037112 m k = 8820 N/m target height = 1.057112 m target speed = 1.0 m/s m = 60.4120 kg g = 5.900428 m/s^2 E = 444.778054 J : Subsystem
  Alpha Target to Leg Length and Leg Angle : MATLAB Function  TreatAsAtomicUnit=on
  AlphaRef : Gain
  Avoid Virtual Leg Length Limits : MATLAB Function  TreatAsAtomicUnit=on
  Avoid Virtual Leg Length Limits1 : MATLAB Function  TreatAsAtomicUnit=on
  Clock : Clock
  Compare To Constant : simulink/Logic and Bit Operations/Compare To Constant  relop=>  const=0  OutDataTypeStr=boolean  ZeroCross=off
  Demux : Demux  Outputs=6
  Demux1 : Demux  Outputs=2
  Demux2 : Demux  Outputs=2
  Demux3 : Demux  Outputs=2
  Detect Fall Nonpositive : simulink/Logic and Bit Operations/Detect Fall Nonpositive  vinit=0  InputProcessing=Inherited  OutDataTypeStr=boolean
  Mux1 : Mux  Inputs=6
  Mux2 : Mux  Inputs=3
  Mux3 : Mux  Inputs=3
  Mux4 : Mux  Inputs=6
  Retracted Leg Trajectory : MATLAB Function  TreatAsAtomicUnit=on
  Sum1 : Sum  Inputs=|+-
  Switch : Switch  Criteria=u2 ~= 0
  Terminator5 : Terminator
  Leg Length Target [m m/s m/s^2] : Outport
  Leg Angle Target [rad rad/s rad/s^2] : Outport  Port=2
  wires:
  Leg Length [m m/s]/1 -> Demux2/1
  Leg Angle [rad rad/s]/1 -> Demux3/1
  Demux3/2 -> Retracted Leg Trajectory/11(dphi_measured)
  Demux3/1 -> Retracted Leg Trajectory/10(phi_measured)
  Demux2/2 -> Retracted Leg Trajectory/9(dl_measured)
  Demux2/1 -> Retracted Leg Trajectory/8(l_measured)
  Retracted Leg Trajectory/6(ddphi) -> Mux1/6
  Alpha Target Law l0 = 1.037112 m k = 8820 N/m target height = 1.057112 m target speed = 1.0 m/s m = 60.4120 kg g = 5.900428 m/s^2 E = 444.778054 J/2(dAlphaRef(t) [rad/s]) -> Alpha Target to Leg Length and Leg Angle/2(dalpha_v)
  Alpha Target Law l0 = 1.037112 m k = 8820 N/m target height = 1.057112 m target speed = 1.0 m/s m = 60.4120 kg g = 5.900428 m/s^2 E = 444.778054 J/3(ddAlphaRef(t) [rad/s^2]) -> Alpha Target to Leg Length and Leg Angle/3(ddalpha_v)
  Mux4/1 -> Switch/1
  Demux1/2 -> Alpha Target to Leg Length and Leg Angle/5(dtheta)
  Demux1/1 -> Alpha Target to Leg Length and Leg Angle/4(theta)
  Demux/1 -> Mux2/1
  Demux/2 -> Mux2/2
  Demux/3 -> Mux2/3
  Demux/4 -> Mux3/1
  Demux/5 -> Mux3/2
  Demux/6 -> Mux3/3
  Mux3/1 -> Leg Angle Target [rad rad/s rad/s^2]/1
  Mux2/1 -> Leg Length Target [m m/s m/s^2]/1
  Switch/1 -> Demux/1
  Avoid Virtual Leg Length Limits/1(l_leg_cmd) -> Retracted Leg Trajectory/4(l_apex), Mux4/1
  Avoid Virtual Leg Length Limits/2(dl_leg_cmd) -> Retracted Leg Trajectory/5(dl_apex), Mux4/2
  Alpha Target to Leg Length and Leg Angle/6(ddphi) -> Mux4/6
  Alpha Target to Leg Length and Leg Angle/5(dphi) -> Retracted Leg Trajectory/7(dphi_apex), Mux4/5
  Avoid Virtual Leg Length Limits/3(ddl_leg_cmd) -> Mux4/3
  Alpha Target to Leg Length and Leg Angle/4(phi) -> Retracted Leg Trajectory/6(phi_apex), Mux4/4
  Detect Fall Nonpositive/1 -> Retracted Leg Trajectory/1(start)
  Retracted Leg Trajectory/5(dphi) -> Mux1/5
  Retracted Leg Trajectory/4(phi) -> Mux1/4
  AlphaRef/1 -> Terminator5/1
  Sum1/1 -> Compare To Constant/1, Alpha Target Law l0 = 1.037112 m k = 8820 N/m target height = 1.057112 m target speed = 1.0 m/s m = 60.4120 kg g = 5.900428 m/s^2 E = 444.778054 J/1(tFall [s])
  Alpha Target Law l0 = 1.037112 m k = 8820 N/m target height = 1.057112 m target speed = 1.0 m/s m = 60.4120 kg g = 5.900428 m/s^2 E = 444.778054 J/1(AlphaRef(t) [rad]) -> Alpha Target to Leg Length and Leg Angle/1(alpha_v), AlphaRef/1
  Clock/1 -> Retracted Leg Trajectory/2(t_system), Sum1/1
  Apex Time [s]/1 -> Retracted Leg Trajectory/3(t_apex), Sum1/2
  Compare To Constant/1 -> Switch/2
  Mux1/1 -> Switch/3
  Torso Pitch [rad rad/s]/1 -> Demux1/1
  Escape [1/0]/1 -> Detect Fall Nonpositive/1
  Alpha Target to Leg Length and Leg Angle/1(l) -> Avoid Virtual Leg Length Limits/1(l_leg_desired)
  Alpha Target to Leg Length and Leg Angle/2(dl) -> Avoid Virtual Leg Length Limits/2(dl_leg_desired)
  Alpha Target to Leg Length and Leg Angle/3(ddl) -> Avoid Virtual Leg Length Limits/3(ddl_leg_desired)
  Avoid Virtual Leg Length Limits1/1(l_leg_cmd) -> Mux1/1
  Avoid Virtual Leg Length Limits1/2(dl_leg_cmd) -> Mux1/2
  Avoid Virtual Leg Length Limits1/3(ddl_leg_cmd) -> Mux1/3
  Retracted Leg Trajectory/1(l) -> Avoid Virtual Leg Length Limits1/1(l_leg_desired)
  Retracted Leg Trajectory/2(dl) -> Avoid Virtual Leg Length Limits1/2(dl_leg_desired)
  Retracted Leg Trajectory/3(ddl) -> Avoid Virtual Leg Length Limits1/3(ddl_leg_desired)

== system spring_mass_model_01/Control/Behavior Control/Primary Leg Behavior/SMM 01/Primary Stance Phase/Virtual Leg Force and Swing Leg Retraction/Hold Initial ==
  in : Inport
  Trigger : TriggerPort  ShowOutputPort=on  PortDimensions=1
  Subsystem : Subsystem
  out : Outport  InitialOutput=[l0_virtual]
  wires:
  in/1 -> Subsystem/1(in)
  Subsystem/1(out) -> out/1
  Trigger/1 -> Subsystem/Enable

== system spring_mass_model_01/Control/Behavior Control/Primary Leg Behavior/SMM 01/Primary Stance Phase/Virtual Leg Force and Swing Leg Retraction/Leg Force-Torque Distribution ==
  Front Spring Torque [Nm] : Inport
  Back Spring Torque [Nm] : Inport  Port=2
  w [m] : Inport  Port=3
  Divide : Product  Inputs=*/
  Sum2 : Sum  Inputs=+|+
  Sum5 : Sum  Inputs=+|-
  Leg Force [N] : Outport
  Leg Torque [Nm] : Outport  Port=2
  wires:
  Divide/1 -> Leg Force [N]/1
  Front Spring Torque [Nm]/1 -> Sum2/1, Sum5/1
  w [m]/1 -> Divide/2
  Sum5/1 -> Divide/1
  Back Spring Torque [Nm]/1 -> Sum2/2, Sum5/2
  Sum2/1 -> Leg Torque [Nm]/1

== system spring_mass_model_01/Control/Behavior Control/Primary Leg Behavior/SMM 01/Primary Stance Phase/Virtual Leg Force and Swing Leg Retraction/Touch Down Trigger ==
  Flight [1/0] : Inport
  Compare To Constant : simulink/Logic and Bit Operations/Compare To Constant  relop=>  const=l0_min_flight_time  OutDataTypeStr=boolean
  Data Type Conversion1 : DataTypeConversion  OutDataTypeStr=boolean
  Logical Operator : Logic  Operator=NOT  IconShape=distinctive  AllPortsSameDT=off  OutDataTypeStr=boolean
  Logical Operator4 : Logic  IconShape=distinctive  AllPortsSameDT=off  OutDataTypeStr=boolean
  S-R Flip-Flop : simulink_extras/Flip Flops/S-R Flip-Flop  initial_condition=0
  Timer : Subsystem
  Trigger [1/0] : Outport
  wires:
  Data Type Conversion1/1 -> S-R Flip-Flop/2
  Flight [1/0]/1 -> Logical Operator/1, Timer/Enable, Data Type Conversion1/1
  Logical Operator4/1 -> S-R Flip-Flop/1
  Logical Operator/1 -> Logical Operator4/1
  Timer/1(timer [s]) -> Compare To Constant/1
  S-R Flip-Flop/1 -> Trigger [1/0]/1
  Compare To Constant/1 -> Logical Operator4/2

== system spring_mass_model_01/Control/Behavior Control/Primary Leg Behavior/SMM 01/Primary Swing Phase/Back//Front Motor PD/Friction Compensation ==
  Right/Left [1/0] : Inport
  Commanded Velocity [rad/s] [back front] : Inport  Port=2
  Product : Product
  Sign : Signum
  Sum1 : Sum
  Switch : Switch  Criteria=u2 ~= 0
  Switch1 : Switch  Criteria=u2 ~= 0
  coulomb_friction_left : Constant  Value=sea_coulomb_friction(3:4)
  coulomb_friction_right : Constant  Value=sea_coulomb_friction(1:2)
  offset_friction_left : Constant  Value=sea_offset_friction(3:4)
  offset_friction_right : Constant  Value=sea_offset_friction(1:2)
  Friction Compensation [Nm] : Outport
  wires:
  Sign/1 -> Product/1
  Switch1/1 -> Product/2
  coulomb_friction_left/1 -> Switch1/3
  coulomb_friction_right/1 -> Switch1/1
  offset_friction_left/1 -> Switch/3
  offset_friction_right/1 -> Switch/1
  Right/Left [1/0]/1 -> Switch/2, Switch1/2
  Product/1 -> Sum1/1
  Sum1/1 -> Friction Compensation [Nm]/1
  Switch/1 -> Sum1/2
  Commanded Velocity [rad/s] [back front]/1 -> Sign/1
